simulink subsystem "PvtSubSys_LSM"  (R2020b)
settings: Solver=VariableStepAuto  StartTime=0.0  StopTime=10.0  RelTol=1e-3
values from neighbouring files (symbols this model uses):
  P_LSM_ALC_Enable = 0.0    [LSM_Parameter.sldd]
  P_LSM_DOP_C0_EN_Limit = 0.8    [LSM_Parameter.sldd]
  P_LSM_DOP_C0_out_Limit = 2.0    [LSM_Parameter.sldd]
  P_LSM_DOP_C1_EN_Limit : value not decoded    [LSM_Parameter.sldd]
  P_LSM_DOP_C1_out_Limit : value not decoded    [LSM_Parameter.sldd]
  P_LSM_DOP_C1AndC2_Lim_X : value not decoded    [LSM_Parameter.sldd]
  P_LSM_DOP_C2_EN_Limit : value not decoded    [LSM_Parameter.sldd]
  P_LSM_DOP_C2_out_Limit : value not decoded    [LSM_Parameter.sldd]
  P_LSM_DOP_In_Pre2Dop_Dis = 1.0    [LSM_Parameter.sldd]
  P_LSM_DOP_Out_Pre2Dop_Dis = 2.0    [LSM_Parameter.sldd]
  P_LSM_DOP_PreDis_X : value not decoded    [LSM_Parameter.sldd]
  P_LSM_DOP_PreDis_Y : value not decoded    [LSM_Parameter.sldd]
  P_LSM_DOPValid_CheckTime = 0.06    [LSM_Parameter.sldd]
  P_LSM_DoubleLine_Curr2Cent_Dislimit = 0.5    [LSM_Parameter.sldd]
  P_LSM_DoubleLine_Dop2Cent_Dislimit = 0.5    [LSM_Parameter.sldd]
  P_LSM_DoubleLine_DOPOut_C1 : value not decoded    [LSM_Parameter.sldd]
  P_LSM_DoubleLine_Pre2Cent_Dislimit = 1.0    [LSM_Parameter.sldd]
  P_LSM_IFV2CenterAxis = 0.0    [LSM_Parameter.sldd]
  P_LSM_IFV2RearAxis = 0.0    [LSM_Parameter.sldd]
  P_LSM_LineSTD_Limit = 0.15    [LSM_Parameter.sldd]
  P_LSM_NOH_Switch = 0.0    [LSM_Parameter.sldd]
  P_LSM_Pre_t = 0.0    [LSM_Parameter.sldd]
  P_LSM_SingleLine_Cent2Edge_Dislimit = 100.0    [LSM_Parameter.sldd]
  P_LSM_SingleLine_Curr2Cent_Dislimit = 0.2    [LSM_Parameter.sldd]
  P_LSM_SingleLine_Dop2Cent_Dislimit = 0.2    [LSM_Parameter.sldd]
  P_LSM_SingleLine_DOPOut_C1 : value not decoded    [LSM_Parameter.sldd]
  P_LSM_SingleLine_Pre2Cent_Dislimit = 0.5    [LSM_Parameter.sldd]
undefined symbols (not defined in the file or in its folder): P_LSM_LineWijCal_C12, P_LSM_LineWijCal_C13, P_LSM_PosLineLcFac
libraries: simulink x92, TrueDurationTime x2
(part 9 of 9)

== matlab function PvtSubSys_LSM/Subsystem/TargetLineCalc_20ms/LALine ==
  data: LA_Count input; L1Conf output uint8 size=1; L1C0 output single size=1; L1C1 output single size=1; L1C2 output single size=1; L1C3 output single size=1; L1DxMin output single size=1; L1DxMax output single size=1; L1A0 input single size=1; L1A1 input single size=1; L1A2 input single size=1; L1A3 input single size=1; L1RaMin input single size=1; L1RaMax input single size=1; L1Avail input uint8 size=1; L1LineType input uint8 size=1; L1DLType input uint8 size=1; L1SideType input uint8 size=1; L1Wid input single size=1; L1Confidence input; L2A0 input single size=1; L2A1 input single size=1; L2A2 input single size=1; L2A3 input single size=1; L2RaMin input single size=1; L2RaMax input single size=1; L2Avail input uint8 size=1; L2LineType input uint8 size=1; L2DLType input uint8 size=1; L2SideType input uint8 size=1; L2Wid input single size=1; L2Confidence input; L3A0 input single size=1; L3A1 input single size=1; L3A2 input single size=1; L3A3 input single size=1; L3RaMin input single size=1; L3RaMax input single size=1; L3Avail input uint8 size=1; L3LineType input uint8 size=1; L3DLType input uint8 size=1; L3SideType input uint8 size=1; L3Wid input single size=1; L3Confidence input; L4A0 input single size=1; L4A1 input single size=1; L4A2 input single size=1; L4A3 input single size=1; L4RaMin input single size=1; L4RaMax input single size=1; L4Avail input uint8 size=1; L4LineType input uint8 size=1; L4DLType input uint8 size=1; L4SideType input uint8 size=1; L4Wid input single size=1; L1Type output uint8 size=1; L1DLM output uint8 size=1; L1Width output single size=1; L1Reliable output; L2Conf output uint8 size=1; L2C0 output single size=1; L2C1 output single size=1; L2C2 output single size=1; L2C3 output single size=1; L2DxMin output single size=1; L2DxMax output single size=1; L2Type output uint8 size=1; L2DLM output uint8 size=1; L2Width output single size=1; L2Reliable output; L3Conf output uint8 size=1; L3C0 output single size=1; L3C1 output single size=1; L3C2 output single size=1; L3C3 output single size=1; L3DxMin output single size=1; L3DxMax output single size=1; L3Type output uint8 size=1; L3DLM output uint8 size=1; L3Width output single size=1; L3Reliable output; L4Conf output uint8 size=1; L4C0 output single size=1; L4C1 output single size=1; L4C2 output single size=1; L4C3 output single size=1; L4DxMin output single size=1; L4DxMax output single size=1; L4Type output uint8 size=1; L4DLM output uint8 size=1; L4Width output single size=1; L4Confidence input; L4Reliable output
function [L1Conf,L1C0,L1C1,L1C2,L1C3,L1DxMin,L1DxMax,L1Type,L1DLM,L1Width,L1Reliable,...
    L2Conf,L2C0,L2C1,L2C2,L2C3,L2DxMin,L2DxMax,L2Type,L2DLM,L2Width,L2Reliable,...
    L3Conf,L3C0,L3C1,L3C2,L3C3,L3DxMin,L3DxMax,L3Type,L3DLM,L3Width,L3Reliable,...
    L4Conf,L4C0,L4C1,L4C2,L4C3,L4DxMin,L4DxMax,L4Type,L4DLM,L4Width,L4Reliable]...
    = LA(LA_Count,L1A0,L1A1,L1A2,L1A3,L1RaMin,L1RaMax,L1Avail,L1LineType,L1DLType,L1SideType,L1Wid,L1Confidence,...
    L2A0,L2A1,L2A2,L2A3,L2RaMin,L2RaMax,L2Avail,L2LineType,L2DLType,L2SideType,L2Wid,L2Confidence,...
    L3A0,L3A1,L3A2,L3A3,L3RaMin,L3RaMax,L3Avail,L3LineType,L3DLType,L3SideType,L3Wid,L3Confidence,...
    L4A0,L4A1,L4A2,L4A3,L4RaMin,L4RaMax,L4Avail,L4LineType,L4DLType,L4SideType,L4Wid,L4Confidence)

L1Conf = uint8(0);
L1C0 = single(0);
L1C1 = single(0);
L1C2 = single(0);
L1C3 = single(0);
L1DxMin = single(0);
L1DxMax = single(0);
L1Type = uint8(0);
L1DLM = uint8(0);
L1Width = single(0);
L1Reliable = single(0);

L2Conf = uint8(0);
L2C0 = single(0);
L2C1 = single(0);
L2C2 = single(0);
L2C3 = single(0);
L2DxMin = single(0);
L2DxMax = single(0);
L2Type = uint8(0);
L2DLM = uint8(0);
L2Width = single(0);
L2Reliable = single(0);

L3Conf = uint8(0);
L3C0 = single(0);
L3C1 = single(0);
L3C2 = single(0);
L3C3 = single(0);
L3DxMin = single(0);
L3DxMax = single(0);
L3Type = uint8(0);
L3DLM = uint8(0);
L3Width = single(0);
L3Reliable = single(0);

L4Conf = uint8(0);
L4C0 = single(0);
L4C1 = single(0);
L4C2 = single(0);
L4C3 = single(0);
L4DxMin = single(0);
L4DxMax = single(0);
L4Type = uint8(0);
L4DLM = uint8(0);
L4Width = single(0);
L4Reliable = single(0);
%%  临车道车道线预处理
if LA_Count >= 1                                     %临车道车道线数量
    if L1SideType==1                                 %左左车道线
        L1Conf = L1Avail;
        L1C0 = L1A0;
        L1C1 = L1A1;
        L1C2 = L1A2;
        L1C3 = L1A3;
        L1DxMin = L1RaMin;
        L1DxMax = L1RaMax;
        L1Type = L1LineType;
        L1DLM = L1DLType;
        L1Width = L1Wid;
        L1Reliable = L1Confidence;
    elseif L1SideType==2                             %左车道右侧车道线
        L2Conf = L1Avail;
        L2C0 = L1A0;
        L2C1 = L1A1;
        L2C2 = L1A2;
        L2C3 = L1A3;
        L2DxMin = L1RaMin;
        L2DxMax = L1RaMax;
        L2Type = L1LineType;
        L2DLM = L1DLType;
        L2Width = L1Wid;
        L2Reliable = L1Confidence;
    elseif L1SideType==3                             %右车道左侧车道线
        L3Conf = L1Avail;
        L3C0 = L1A0;
        L3C1 = L1A1;
        L3C2 = L1A2;
        L3C3 = L1A3;
        L3DxMin = L1RaMin;
        L3DxMax = L1RaMax;
        L3Type = L1LineType;
        L3DLM = L1DLType;
        L3Width = L1Wid;
        L3Reliable = L1Confidence;
    elseif L1SideType==4                             %右右车道线
        L4Conf = L1Avail;
        L4C0 = L1A0;
        L4C1 = L1A1;
        L4C2 = L1A2;
        L4C3 = L1A3;
        L4DxMin = L1RaMin;
        L4DxMax = L1RaMax;
        L4Type = L1LineType;
        L4DLM = L1DLType;
        L4Width = L1Wid;
        L4Reliable = L1Confidence;
    end
    if LA_Count >= 2
        if L2SideType==1
            L1Conf = L2Avail;
            L1C0 = L2A0;
            L1C1 = L2A1;
            L1C2 = L2A2;
            L1C3 = L2A3;
            L1DxMin = L2RaMin;
            L1DxMax = L2RaMax;
            L1Type = L2LineType;
            L1DLM = L2DLType;
            L1Width = L2Wid;
            L1Reliable = L2Confidence;
        elseif L2SideType==2
            L2Conf = L2Avail;
            L2C0 = L2A0;
            L2C1 = L2A1;
            L2C2 = L2A2;
            L2C3 = L2A3;
            L2DxMin = L2RaMin;
            L2DxMax = L2RaMax;
            L2Type = L2LineType;
            L2DLM = L2DLType;
            L2Width = L2Wid;
            L2Reliable = L2Confidence;
        elseif L2SideType==3
            L3Conf = L2Avail;
            L3C0 = L2A0;
            L3C1 = L2A1;
            L3C2 = L2A2;
            L3C3 = L2A3;
            L3DxMin = L2RaMin;
            L3DxMax = L2RaMax;
            L3Type = L2LineType;
            L3DLM = L2DLType;
            L3Width = L2Wid;
            L3Reliable = L2Confidence;
        elseif L2SideType==4
            L4Conf = L2Avail;
            L4C0 = L2A0;
            L4C1 = L2A1;
            L4C2 = L2A2;
            L4C3 = L2A3;
            L4DxMin = L2RaMin;
            L4DxMax = L2RaMax;
            L4Type = L2LineType;
            L4DLM = L2DLType;
            L4Width = L2Wid;
            L4Reliable = L2Confidence;
        end
        if LA_Count >= 3
            if L3SideType==1
                L1Conf = L3Avail;
                L1C0 = L3A0;
                L1C1 = L3A1;
                L1C2 = L3A2;
                L1C3 = L3A3;
                L1DxMin = L3RaMin;
                L1DxMax = L3RaMax;
                L1Type = L3LineType;
                L1DLM = L3DLType;
                L1Width = L3Wid;
                L1Reliable = L3Confidence;
            elseif L3SideType==2
                L2Conf = L3Avail;
                L2C0 = L3A0;
                L2C1 = L3A1;
                L2C2 = L3A2;
                L2C3 = L3A3;
                L2DxMin = L3RaMin;
                L2DxMax = L3RaMax;
                L2Type = L3LineType;
                L2DLM = L3DLType;
                L2Width = L3Wid;
                L2Reliable = L3Confidence;
            elseif L3SideType==3
                L3Conf = L3Avail;
                L3C0 = L3A0;
                L3C1 = L3A1;
                L3C2 = L3A2;
                L3C3 = L3A3;
                L3DxMin = L3RaMin;
                L3DxMax = L3RaMax;
                L3Type = L3LineType;
                L3DLM = L3DLType;
                L3Width = L3Wid;
                L3Reliable = L3Confidence;
            elseif L3SideType==4
                L4Conf = L3Avail;
                L4C0 = L3A0;
                L4C1 = L3A1;
                L4C2 = L3A2;
                L4C3 = L3A3;
                L4DxMin = L3RaMin;
                L4DxMax = L3RaMax;
                L4Type = L3LineType;
                L4DLM = L3DLType;
                L4Width = L3Wid;
                L4Reliable = L3Confidence;
            end
            if LA_Count >= 4
                if L4SideType==1
                    L1Conf = L4Avail;
                    L1C0 = L4A0;
                    L1C1 = L4A1;
                    L1C2 = L4A2;
                    L1C3 = L4A3;
                    L1DxMin = L4RaMin;
                    L1DxMax = L4RaMax;
                    L1Type = L4LineType;
                    L1DLM = L4DLType;
                    L1Width = L4Wid;
                    L1Reliable = L4Confidence;
                elseif L4SideType==2
                    L2Conf = L4Avail;
                    L2C0 = L4A0;
                    L2C1 = L4A1;
                    L2C2 = L4A2;
                    L2C3 = L4A3;
                    L2DxMin = L4RaMin;
                    L2DxMax = L4RaMax;
                    L2Type = L4LineType;
                    L2DLM = L4DLType;
                    L2Width = L4Wid;
                    L2Reliable = L4Confidence;
                elseif L4SideType==3
                    L3Conf = L4Avail;
                    L3C0 = L4A0;
                    L3C1 = L4A1;
                    L3C2 = L4A2;
                    L3C3 = L4A3;
                    L3DxMin = L4RaMin;
                    L3DxMax = L4RaMax;
                    L3Type = L4LineType;
                    L3DLM = L4DLType;
                    L3Width = L4Wid;
                    L3Reliable = L4Confidence;
                elseif L4SideType==4
                    L4Conf = L4Avail;
                    L4C0 = L4A0;
                    L4C1 = L4A1;
                    L4C2 = L4A2;
                    L4C3 = L4A3;
                    L4DxMin = L4RaMin;
                    L4DxMax = L4RaMax;
                    L4Type = L4LineType;
                    L4DLM = L4DLType;
                    L4Width = L4Wid;
                    L4Reliable = L4Confidence;
                end
            end
        end
    end
end
